simulink model "SMC_Controller"  (R2025a)
settings: Solver=VariableStepAuto  StartTime=0.0  StopTime=10.0  RelTol=1e-3
settings Model: Creator=xing2  LastModifiedBy=xing2

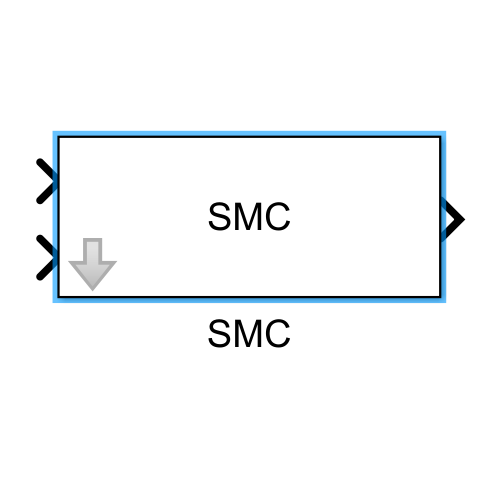
[thumbnail: Simulink's stored preview of the top-level diagram]
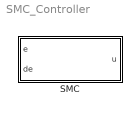
== system SMC_Controller ==
  SMC : Subsystem  mask{lambda=10, K_smc=3, phi=0.1}
      mask prompts: lambda "lambda (slope)"; K_smc "K (gain)"; phi "phi (boundary)"
      mask help: Sliding Mode Controller with boundary layer
      mask Display: disp('SMC');

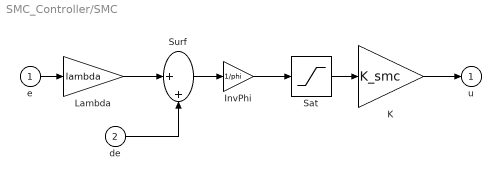
== system SMC_Controller/SMC ==
  e : Inport
  de : Inport  Port=2
  InvPhi : Gain  Gain=1/phi
  K : Gain  Gain=K_smc
  Lambda : Gain  Gain=lambda
  Sat : Saturate  UpperLimit=1  LowerLimit=-1
  Surf : Sum  Inputs=|++
  u : Outport
  wires:
  e/1 -> Lambda/1
  Sat/1 -> K/1
  Lambda/1 -> Surf/1
  InvPhi/1 -> Sat/1
  de/1 -> Surf/2
  K/1 -> u/1
  Surf/1 -> InvPhi/1
